simulink library "BechamoNasaOpenModels"  (R2024b)
settings: Solver=VariableStepAuto  StartTime=0.0  StopTime=10.0  RelTol=1e-3
values from neighbouring files (symbols this model uses):
  Cl_aileron_wing_1 = Cl_mat.Claileron_wing.axes1.value    [setupMavrik.m]
  Cl_aileron_wing_2 = Cl_mat.Claileron_wing.axes2.value    [setupMavrik.m]
  Cl_aileron_wing_3 = Cl_mat.Claileron_wing.axes3.value    [setupMavrik.m]
  Cl_aileron_wing_val = Cl_mat.Claileron_wing.value    [setupMavrik.m]
  Cl_elevator_tail_1 = Cl_mat.Clelevator_tail.axes1.value    [setupMavrik.m]
  Cl_elevator_tail_2 = Cl_mat.Clelevator_tail.axes2.value    [setupMavrik.m]
  Cl_elevator_tail_3 = Cl_mat.Clelevator_tail.axes3.value    [setupMavrik.m]
  Cl_elevator_tail_val = Cl_mat.Clelevator_tail.value    [setupMavrik.m]
  Cl_flap_wing_1 = Cl_mat.Clflap_wing.axes1.value    [setupMavrik.m]
  Cl_flap_wing_2 = Cl_mat.Clflap_wing.axes2.value    [setupMavrik.m]
  Cl_flap_wing_3 = Cl_mat.Clflap_wing.axes3.value    [setupMavrik.m]
  Cl_flap_wing_val = Cl_mat.Clflap_wing.value    [setupMavrik.m]
  Cl_hover_fuse_1 = Cl_mat.Clhover_fuse.axes1.value    [setupMavrik.m]
  Cl_hover_fuse_2 = Cl_mat.Clhover_fuse.axes2.value    [setupMavrik.m]
  Cl_hover_fuse_3 = Cl_mat.Clhover_fuse.axes3.value    [setupMavrik.m]
  Cl_hover_fuse_val = Cl_mat.Clhover_fuse.value    [setupMavrik.m]
  Cl_rudder_tail_1 = Cl_mat.Clrudder_tail.axes1.value    [setupMavrik.m]
  Cl_rudder_tail_2 = Cl_mat.Clrudder_tail.axes2.value    [setupMavrik.m]
  Cl_rudder_tail_3 = Cl_mat.Clrudder_tail.axes3.value    [setupMavrik.m]
  Cl_rudder_tail_val = Cl_mat.Clrudder_tail.value    [setupMavrik.m]
  Cl_tail_1 = Cl_mat.Cltail.axes1.value    [setupMavrik.m]
  Cl_tail_2 = Cl_mat.Cltail.axes2.value    [setupMavrik.m]
  Cl_tail_3 = Cl_mat.Cltail.axes3.value    [setupMavrik.m]
  Cl_tail_damp_p_1 = Cl_mat.Cltail_damp_p.axes1.value    [setupMavrik.m]
  Cl_tail_damp_p_2 = Cl_mat.Cltail_damp_p.axes2.value    [setupMavrik.m]
  Cl_tail_damp_p_3 = Cl_mat.Cltail_damp_p.axes3.value    [setupMavrik.m]
  Cl_tail_damp_p_val = Cl_mat.Cltail_damp_p.value    [setupMavrik.m]
  Cl_tail_damp_q_1 = Cl_mat.Cltail_damp_q.axes1.value    [setupMavrik.m]
  Cl_tail_damp_q_2 = Cl_mat.Cltail_damp_q.axes2.value    [setupMavrik.m]
  Cl_tail_damp_q_3 = Cl_mat.Cltail_damp_q.axes3.value    [setupMavrik.m]
  Cl_tail_damp_q_val = Cl_mat.Cltail_damp_q.value    [setupMavrik.m]
  Cl_tail_damp_r_1 = Cl_mat.Cltail_damp_r.axes1.value    [setupMavrik.m]
  Cl_tail_damp_r_2 = Cl_mat.Cltail_damp_r.axes2.value    [setupMavrik.m]
  Cl_tail_damp_r_3 = Cl_mat.Cltail_damp_r.axes3.value    [setupMavrik.m]
  Cl_tail_damp_r_val = Cl_mat.Cltail_damp_r.value    [setupMavrik.m]
  Cl_tail_val = Cl_mat.Cltail.value    [setupMavrik.m]
  Cl_wing_1 = Cl_mat.Clwing.axes1.value    [setupMavrik.m]
  Cl_wing_2 = Cl_mat.Clwing.axes2.value    [setupMavrik.m]
  Cl_wing_3 = Cl_mat.Clwing.axes3.value    [setupMavrik.m]
  Cl_wing_damp_p_1 = Cl_mat.Clwing_damp_p.axes1.value    [setupMavrik.m]
  Cl_wing_damp_p_2 = Cl_mat.Clwing_damp_p.axes2.value    [setupMavrik.m]
  Cl_wing_damp_p_3 = Cl_mat.Clwing_damp_p.axes3.value    [setupMavrik.m]
  Cl_wing_damp_p_val = Cl_mat.Clwing_damp_p.value    [setupMavrik.m]
  Cl_wing_damp_q_1 = Cl_mat.Clwing_damp_q.axes1.value    [setupMavrik.m]
  Cl_wing_damp_q_2 = Cl_mat.Clwing_damp_q.axes2.value    [setupMavrik.m]
  Cl_wing_damp_q_3 = Cl_mat.Clwing_damp_q.axes3.value    [setupMavrik.m]
  Cl_wing_damp_q_val = Cl_mat.Clwing_damp_q.value    [setupMavrik.m]
  Cl_wing_damp_r_1 = Cl_mat.Clwing_damp_r.axes1.value    [setupMavrik.m]
  Cl_wing_damp_r_2 = Cl_mat.Clwing_damp_r.axes2.value    [setupMavrik.m]
  Cl_wing_damp_r_3 = Cl_mat.Clwing_damp_r.axes3.value    [setupMavrik.m]
  Cl_wing_damp_r_val = Cl_mat.Clwing_damp_r.value    [setupMavrik.m]
  Cl_wing_val = Cl_mat.Clwing.value    [setupMavrik.m]
  Cm_aileron_wing_1 = Cm_mat.Cmaileron_wing.axes1.value    [setupMavrik.m]
  Cm_aileron_wing_2 = Cm_mat.Cmaileron_wing.axes2.value    [setupMavrik.m]
  Cm_aileron_wing_3 = Cm_mat.Cmaileron_wing.axes3.value    [setupMavrik.m]
  Cm_aileron_wing_val = Cm_mat.Cmaileron_wing.value    [setupMavrik.m]
  Cm_elevator_tail_1 = Cm_mat.Cmelevator_tail.axes1.value    [setupMavrik.m]
  Cm_elevator_tail_2 = Cm_mat.Cmelevator_tail.axes2.value    [setupMavrik.m]
  Cm_elevator_tail_3 = Cm_mat.Cmelevator_tail.axes3.value    [setupMavrik.m]
  Cm_elevator_tail_val = Cm_mat.Cmelevator_tail.value    [setupMavrik.m]
  Cm_flap_wing_1 = Cm_mat.Cmflap_wing.axes1.value    [setupMavrik.m]
  Cm_flap_wing_2 = Cm_mat.Cmflap_wing.axes2.value    [setupMavrik.m]
  Cm_flap_wing_3 = Cm_mat.Cmflap_wing.axes3.value    [setupMavrik.m]
  Cm_flap_wing_val = Cm_mat.Cmflap_wing.value    [setupMavrik.m]
  Cm_hover_fuse_1 = Cm_mat.Cmhover_fuse.axes1.value    [setupMavrik.m]
  Cm_hover_fuse_2 = Cm_mat.Cmhover_fuse.axes2.value    [setupMavrik.m]
  Cm_hover_fuse_3 = Cm_mat.Cmhover_fuse.axes3.value    [setupMavrik.m]
  Cm_hover_fuse_val = Cm_mat.Cmhover_fuse.value    [setupMavrik.m]
  Cm_rudder_tail_1 = Cm_mat.Cmrudder_tail.axes1.value    [setupMavrik.m]
  Cm_rudder_tail_2 = Cm_mat.Cmrudder_tail.axes2.value    [setupMavrik.m]
  Cm_rudder_tail_3 = Cm_mat.Cmrudder_tail.axes3.value    [setupMavrik.m]
  Cm_rudder_tail_val = Cm_mat.Cmrudder_tail.value    [setupMavrik.m]
  Cm_tail_1 = Cm_mat.Cmtail.axes1.value    [setupMavrik.m]
  Cm_tail_2 = Cm_mat.Cmtail.axes2.value    [setupMavrik.m]
  Cm_tail_3 = Cm_mat.Cmtail.axes3.value    [setupMavrik.m]
  Cm_tail_damp_p_1 = Cm_mat.Cmtail_damp_p.axes1.value    [setupMavrik.m]
  Cm_tail_damp_p_2 = Cm_mat.Cmtail_damp_p.axes2.value    [setupMavrik.m]
  Cm_tail_damp_p_3 = Cm_mat.Cmtail_damp_p.axes3.value    [setupMavrik.m]
  Cm_tail_damp_p_val = Cm_mat.Cmtail_damp_p.value    [setupMavrik.m]
  Cm_tail_damp_q_1 = Cm_mat.Cmtail_damp_q.axes1.value    [setupMavrik.m]
  Cm_tail_damp_q_2 = Cm_mat.Cmtail_damp_q.axes2.value    [setupMavrik.m]
  Cm_tail_damp_q_3 = Cm_mat.Cmtail_damp_q.axes3.value    [setupMavrik.m]
  Cm_tail_damp_q_val = Cm_mat.Cmtail_damp_q.value    [setupMavrik.m]
  Cm_tail_damp_r_1 = Cm_mat.Cmtail_damp_r.axes1.value    [setupMavrik.m]
  Cm_tail_damp_r_2 = Cm_mat.Cmtail_damp_r.axes2.value    [setupMavrik.m]
  Cm_tail_damp_r_3 = Cm_mat.Cmtail_damp_r.axes3.value    [setupMavrik.m]
  Cm_tail_damp_r_val = Cm_mat.Cmtail_damp_r.value    [setupMavrik.m]
  Cm_tail_val = Cm_mat.Cmtail.value    [setupMavrik.m]
  Cm_wing_1 = Cm_mat.Cmwing.axes1.value    [setupMavrik.m]
  Cm_wing_2 = Cm_mat.Cmwing.axes2.value    [setupMavrik.m]
  Cm_wing_3 = Cm_mat.Cmwing.axes3.value    [setupMavrik.m]
  Cm_wing_damp_p_1 = Cm_mat.Cmwing_damp_p.axes1.value    [setupMavrik.m]
  Cm_wing_damp_p_2 = Cm_mat.Cmwing_damp_p.axes2.value    [setupMavrik.m]
  Cm_wing_damp_p_3 = Cm_mat.Cmwing_damp_p.axes3.value    [setupMavrik.m]
  Cm_wing_damp_p_val = Cm_mat.Cmwing_damp_p.value    [setupMavrik.m]
  Cm_wing_damp_q_1 = Cm_mat.Cmwing_damp_q.axes1.value    [setupMavrik.m]
  Cm_wing_damp_q_2 = Cm_mat.Cmwing_damp_q.axes2.value    [setupMavrik.m]
  Cm_wing_damp_q_3 = Cm_mat.Cmwing_damp_q.axes3.value    [setupMavrik.m]
  Cm_wing_damp_q_val = Cm_mat.Cmwing_damp_q.value    [setupMavrik.m]
  Cm_wing_damp_r_1 = Cm_mat.Cmwing_damp_r.axes1.value    [setupMavrik.m]
  Cm_wing_damp_r_2 = Cm_mat.Cmwing_damp_r.axes2.value    [setupMavrik.m]
  Cm_wing_damp_r_3 = Cm_mat.Cmwing_damp_r.axes3.value    [setupMavrik.m]
  Cm_wing_damp_r_val = Cm_mat.Cmwing_damp_r.value    [setupMavrik.m]
  Cm_wing_val = Cm_mat.Cmwing.value    [setupMavrik.m]
  Cn_aileron_wing_1 = Cn_mat.Cnaileron_wing.axes1.value    [setupMavrik.m]
  Cn_aileron_wing_2 = Cn_mat.Cnaileron_wing.axes2.value    [setupMavrik.m]
  Cn_aileron_wing_3 = Cn_mat.Cnaileron_wing.axes3.value    [setupMavrik.m]
  Cn_aileron_wing_val = Cn_mat.Cnaileron_wing.value    [setupMavrik.m]
  Cn_elevator_tail_1 = Cn_mat.Cnelevator_tail.axes1.value    [setupMavrik.m]
  Cn_elevator_tail_2 = Cn_mat.Cnelevator_tail.axes2.value    [setupMavrik.m]
  Cn_elevator_tail_3 = Cn_mat.Cnelevator_tail.axes3.value    [setupMavrik.m]
  Cn_elevator_tail_val = Cn_mat.Cnelevator_tail.value    [setupMavrik.m]
  Cn_flap_wing_1 = Cn_mat.Cnflap_wing.axes1.value    [setupMavrik.m]
  Cn_flap_wing_2 = Cn_mat.Cnflap_wing.axes2.value    [setupMavrik.m]
  Cn_flap_wing_3 = Cn_mat.Cnflap_wing.axes3.value    [setupMavrik.m]
  Cn_flap_wing_val = Cn_mat.Cnflap_wing.value    [setupMavrik.m]
  Cn_hover_fuse_1 = Cn_mat.Cnhover_fuse.axes1.value    [setupMavrik.m]
  Cn_hover_fuse_2 = Cn_mat.Cnhover_fuse.axes2.value    [setupMavrik.m]
  Cn_hover_fuse_3 = Cn_mat.Cnhover_fuse.axes3.value    [setupMavrik.m]
  Cn_hover_fuse_val = Cn_mat.Cnhover_fuse.value    [setupMavrik.m]
  ... (+319 more)
libraries: matrix_library x15, sharedtransform x2, $bdroot x1, shared6dof x1
(part 16 of 19)

== matlab function BechamoNasaOpenModels/Mavrik v1/Mavrik Aero/Kq/MATLAB Function205 ==
  data: u input size=[1 45]; Wing_Transform output
function Wing_Transform = fcn(u)

% Find Interpolation Points
variable_indices = struct('U', 1, 'alpha', 2, 'beta', 3, 'p', 4, 'q', 5, 'r', 6, 'wing_alpha', 7, 'wing_beta', 8, 'wing_RPM', 9, 'left_alpha', 10,...
    'right_alpha', 11, 'left_beta', 12, 'right_beta', 13, 'wing_prop_alpha', 14, 'wing_prop_beta', 15, 'tail_alpha', 16, 'tail_beta', 17, 'tail_RPM', 18, 'tailLeft_alpha', 19, 'tailRight_alpha', 20,...
    'tailLeft_beta', 21, 'tailRight_beta', 22, 'tail_prop_alpha', 23, 'tail_prop_beta', 24, 'Q', 25, 'aileron', 26, 'elevator', 27, 'flap', 28, 'rudder', 29, 'wing_tilt', 30,...
    'tail_tilt', 31, 'RPM_tailLeft', 32, 'RPM_tailRight', 33, 'RPM_leftOut1', 34, 'RPM_left2', 35, 'RPM_left3', 36, 'RPM_left4', 37, 'RPM_left5', 38, 'RPM_left6In', 39, 'RPM_right7In', 40,...
    'RPM_right8', 41, 'RPM_right9', 42, 'RPM_right10', 43, 'RPM_right11', 44, 'RPM_right12Out', 45);

wing_tilt = u(variable_indices.wing_tilt);
Wing_Transform = [cos(wing_tilt) 0 sin(wing_tilt); 0 1 0; -sin(wing_tilt) 0 cos(wing_tilt)];

end

% y = [U, alpha, beta, p, q, r, wing_alpha, wing_beta, wing_RPM, left_alpha, right_alpha, left_beta, right_beta, wing_prop_alpha, wing_prop_beta, ...
    % tail_alpha, tail_beta, tail_RPM, tailLeft_alpha, tailRight_alpha, tailLeft_beta, tailRight_beta, tail_prop_alpha, ...
    % tail_prop_beta, Q, aileron, elevator, flap, rudder, wing_tilt, tail_tilt, RPM_tailLeft, RPM_tailRight, RPM_leftOut1, RPM_left2, ...
    % RPM_left3, RPM_left4, RPM_left5, RPM_left6In, RPM_right7In, RPM_right8, RPM_right9, RPM_right10, RPM_right11, RPM_right12Out];

== matlab function BechamoNasaOpenModels/Mavrik v1/Mavrik Aero/Cy/CY_wing_damp_p ==
  data: u input size=[1 45]; interp_point_1 output; interp_point_2 output; interp_point_3 output; interp_point_4 output; interp_point_5 output; interp_point_6 output
function [interp_point_1, interp_point_2, interp_point_3, interp_point_4, interp_point_5, interp_point_6] = fcn(u)

% Find Interpolation Points
variable_indices = struct('U', 1, 'alpha', 2, 'beta', 3, 'p', 4, 'q', 5, 'r', 6, 'wing_alpha', 7, 'wing_beta', 8, 'wing_RPM', 9, 'left_alpha', 10,...
    'right_alpha', 11, 'left_beta', 12, 'right_beta', 13, 'wing_prop_alpha', 14, 'wing_prop_beta', 15, 'tail_alpha', 16, 'tail_beta', 17, 'tail_RPM', 18, 'tailLeft_alpha', 19, 'tailRight_alpha', 20,...
    'tailLeft_beta', 21, 'tailRight_beta', 22, 'tail_prop_alpha', 23, 'tail_prop_beta', 24, 'Q', 25, 'aileron', 26, 'elevator', 27, 'flap', 28, 'rudder', 29, 'wing_tilt', 30,...
    'tail_tilt', 31, 'RPM_tailLeft', 32, 'RPM_tailRight', 33, 'RPM_leftOut1', 34, 'RPM_left2', 35, 'RPM_left3', 36, 'RPM_left4', 37, 'RPM_left5', 38, 'RPM_left6In', 39, 'RPM_right7In', 40,...
    'RPM_right8', 41, 'RPM_right9', 42, 'RPM_right10', 43, 'RPM_right11', 44, 'RPM_right12Out', 45);

interp_point_1  = u(variable_indices.wing_alpha);
interp_point_2  = u(variable_indices.wing_beta);
interp_point_3  = u(variable_indices.U);
interp_point_4  = u(variable_indices.wing_RPM);
interp_point_5  = u(variable_indices.wing_prop_alpha);
interp_point_6  = u(variable_indices.wing_prop_beta);

end

% y = [U, alpha, beta, p, q, r, wing_alpha, wing_beta, wing_RPM, left_alpha, right_alpha, left_beta, right_beta, wing_prop_alpha, wing_prop_beta, ...
    % tail_alpha, tail_beta, tail_RPM, tailLeft_alpha, tailRight_alpha, tailLeft_beta, tailRight_beta, tail_prop_alpha, ...
    % tail_prop_beta, Q, aileron, elevator, flap, rudder, wing_tilt, tail_tilt, RPM_tailLeft, RPM_tailRight, RPM_leftOut1, RPM_left2, ...
    % RPM_left3, RPM_left4, RPM_left5, RPM_left6In, RPM_right7In, RPM_right8, RPM_right9, RPM_right10, RPM_right11, RPM_right12Out];

== matlab function BechamoNasaOpenModels/Mavrik v1/Mavrik Aero/Cy/CY_wing_damp_q ==
  data: u input size=[1 45]; interp_point_1 output; interp_point_2 output; interp_point_3 output; interp_point_4 output; interp_point_5 output; interp_point_6 output
function [interp_point_1, interp_point_2, interp_point_3, interp_point_4, interp_point_5, interp_point_6] = fcn(u)

% Find Interpolation Points
variable_indices = struct('U', 1, 'alpha', 2, 'beta', 3, 'p', 4, 'q', 5, 'r', 6, 'wing_alpha', 7, 'wing_beta', 8, 'wing_RPM', 9, 'left_alpha', 10,...
    'right_alpha', 11, 'left_beta', 12, 'right_beta', 13, 'wing_prop_alpha', 14, 'wing_prop_beta', 15, 'tail_alpha', 16, 'tail_beta', 17, 'tail_RPM', 18, 'tailLeft_alpha', 19, 'tailRight_alpha', 20,...
    'tailLeft_beta', 21, 'tailRight_beta', 22, 'tail_prop_alpha', 23, 'tail_prop_beta', 24, 'Q', 25, 'aileron', 26, 'elevator', 27, 'flap', 28, 'rudder', 29, 'wing_tilt', 30,...
    'tail_tilt', 31, 'RPM_tailLeft', 32, 'RPM_tailRight', 33, 'RPM_leftOut1', 34, 'RPM_left2', 35, 'RPM_left3', 36, 'RPM_left4', 37, 'RPM_left5', 38, 'RPM_left6In', 39, 'RPM_right7In', 40,...
    'RPM_right8', 41, 'RPM_right9', 42, 'RPM_right10', 43, 'RPM_right11', 44, 'RPM_right12Out', 45);

interp_point_1  = u(variable_indices.wing_alpha);
interp_point_2  = u(variable_indices.wing_beta);
interp_point_3  = u(variable_indices.U);
interp_point_4  = u(variable_indices.wing_RPM);
interp_point_5  = u(variable_indices.wing_prop_alpha);
interp_point_6  = u(variable_indices.wing_prop_beta);

end

% y = [U, alpha, beta, p, q, r, wing_alpha, wing_beta, wing_RPM, left_alpha, right_alpha, left_beta, right_beta, wing_prop_alpha, wing_prop_beta, ...
    % tail_alpha, tail_beta, tail_RPM, tailLeft_alpha, tailRight_alpha, tailLeft_beta, tailRight_beta, tail_prop_alpha, ...
    % tail_prop_beta, Q, aileron, elevator, flap, rudder, wing_tilt, tail_tilt, RPM_tailLeft, RPM_tailRight, RPM_leftOut1, RPM_left2, ...
    % RPM_left3, RPM_left4, RPM_left5, RPM_left6In, RPM_right7In, RPM_right8, RPM_right9, RPM_right10, RPM_right11, RPM_right12Out];

== matlab function BechamoNasaOpenModels/Mavrik v1/Mavrik Aero/Function Block 1 ==
  data: u input size=[1 9]; y output size=[1 45]; actuators input
function y  = fcn(u, actuators)

% Setup input states
U = sqrt(u(1)^2+u(2)^2+u(3)^2);
alpha = atan2(u(3), u(1));
beta = atan2(u(2),sqrt(u(1)^2+u(3)^2));
p = u(4);
q = u(5);
r = u(6);
phi = u(7);
theta = u(8);
psi = u(9);

rho = 1.225;

% Actuation Inputs
wing_tilt = actuators(1);
tail_tilt = actuators(2); 
aileron = actuators(3);
elevator = actuators(4);
flap = actuators(5);
rudder = actuators(6);
RPM_tailLeft = actuators(7);
RPM_tailRight = actuators(8);
RPM_leftOut1 = actuators(9);
RPM_left2 = actuators(10);
RPM_left3 = actuators(11);
RPM_left4 = actuators(12);
RPM_left5 = actuators(13);
RPM_left6In = actuators(14);
RPM_right7In = actuators(15);
RPM_right8 = actuators(16);
RPM_right9 = actuators(17);
RPM_right10 = actuators(18);
RPM_right11 = actuators(19);
RPM_right12Out = actuators(20);

% Calculate alpha/beta for local tables

wing_alpha = alpha + wing_tilt;
wing_beta = beta;
wing_RPM = 1/12 * (RPM_leftOut1 + RPM_left2 + RPM_left3 + RPM_left4 + RPM_left5 + RPM_left6In + RPM_right7In + RPM_right8 + RPM_right9 + RPM_right10 + RPM_right11 + RPM_right12Out);
left_alpha = alpha + wing_tilt; 
right_alpha = alpha + wing_tilt;
left_beta = beta;
right_beta = beta;
wing_prop_alpha = 1/2 * sum(left_alpha + right_alpha);
wing_prop_beta = 1/2 * sum(left_beta + right_beta);
tail_alpha = alpha + tail_tilt;
tail_beta = beta;
tail_RPM = 0.5 * (RPM_tailRight + RPM_tailLeft); 
tailLeft_alpha = alpha + tail_tilt;
tailRight_alpha = alpha + tail_tilt; 
tailLeft_beta = beta;
tailRight_beta = beta; 
tail_prop_alpha = 0.5 * (tailLeft_alpha + tailRight_alpha);
tail_prop_beta = 0.5 * (tailLeft_beta + tailRight_beta); 
Q = 0.5*rho*U^2;

y = [U, alpha, beta, p, q, r, wing_alpha, wing_beta, wing_RPM, left_alpha, right_alpha, left_beta, right_beta, wing_prop_alpha, wing_prop_beta, ...
    tail_alpha, tail_beta, tail_RPM, tailLeft_alpha, tailRight_alpha, tailLeft_beta, tailRight_beta, tail_prop_alpha, ...
    tail_prop_beta, Q, aileron, elevator, flap, rudder, wing_tilt, tail_tilt, RPM_tailLeft, RPM_tailRight, RPM_leftOut1, RPM_left2, ...
    RPM_left3, RPM_left4, RPM_left5, RPM_left6In, RPM_right7In, RPM_right8, RPM_right9, RPM_right10, RPM_right11, RPM_right12Out];

end

== matlab function BechamoNasaOpenModels/Mavrik v1/Mavrik Aero/Cy/CY_wing_damp_r ==
  data: u input size=[1 45]; interp_point_1 output; interp_point_2 output; interp_point_3 output; interp_point_4 output; interp_point_5 output; interp_point_6 output
function [interp_point_1, interp_point_2, interp_point_3, interp_point_4, interp_point_5, interp_point_6] = fcn(u)

% Find Interpolation Points
variable_indices = struct('U', 1, 'alpha', 2, 'beta', 3, 'p', 4, 'q', 5, 'r', 6, 'wing_alpha', 7, 'wing_beta', 8, 'wing_RPM', 9, 'left_alpha', 10,...
    'right_alpha', 11, 'left_beta', 12, 'right_beta', 13, 'wing_prop_alpha', 14, 'wing_prop_beta', 15, 'tail_alpha', 16, 'tail_beta', 17, 'tail_RPM', 18, 'tailLeft_alpha', 19, 'tailRight_alpha', 20,...
    'tailLeft_beta', 21, 'tailRight_beta', 22, 'tail_prop_alpha', 23, 'tail_prop_beta', 24, 'Q', 25, 'aileron', 26, 'elevator', 27, 'flap', 28, 'rudder', 29, 'wing_tilt', 30,...
    'tail_tilt', 31, 'RPM_tailLeft', 32, 'RPM_tailRight', 33, 'RPM_leftOut1', 34, 'RPM_left2', 35, 'RPM_left3', 36, 'RPM_left4', 37, 'RPM_left5', 38, 'RPM_left6In', 39, 'RPM_right7In', 40,...
    'RPM_right8', 41, 'RPM_right9', 42, 'RPM_right10', 43, 'RPM_right11', 44, 'RPM_right12Out', 45);

interp_point_1  = u(variable_indices.wing_alpha);
interp_point_2  = u(variable_indices.wing_beta);
interp_point_3  = u(variable_indices.U);
interp_point_4  = u(variable_indices.wing_RPM);
interp_point_5  = u(variable_indices.wing_prop_alpha);
interp_point_6  = u(variable_indices.wing_prop_beta);

end

% y = [U, alpha, beta, p, q, r, wing_alpha, wing_beta, wing_RPM, left_alpha, right_alpha, left_beta, right_beta, wing_prop_alpha, wing_prop_beta, ...
    % tail_alpha, tail_beta, tail_RPM, tailLeft_alpha, tailRight_alpha, tailLeft_beta, tailRight_beta, tail_prop_alpha, ...
    % tail_prop_beta, Q, aileron, elevator, flap, rudder, wing_tilt, tail_tilt, RPM_tailLeft, RPM_tailRight, RPM_leftOut1, RPM_left2, ...
    % RPM_left3, RPM_left4, RPM_left5, RPM_left6In, RPM_right7In, RPM_right8, RPM_right9, RPM_right10, RPM_right11, RPM_right12Out];

== matlab function BechamoNasaOpenModels/Mavrik v1/Mavrik Aero/Cz/CZ_aileron_wing ==
  data: u input size=[1 45]; interp_point_1 output; interp_point_2 output; interp_point_3 output; interp_point_4 output; interp_point_5 output; interp_point_6 output; interp_point_7 output
function [interp_point_1, interp_point_2, interp_point_3, interp_point_4, interp_point_5, interp_point_6, interp_point_7] = fcn(u)

% Find Interpolation Points
variable_indices = struct('U', 1, 'alpha', 2, 'beta', 3, 'p', 4, 'q', 5, 'r', 6, 'wing_alpha', 7, 'wing_beta', 8, 'wing_RPM', 9, 'left_alpha', 10,...
    'right_alpha', 11, 'left_beta', 12, 'right_beta', 13, 'wing_prop_alpha', 14, 'wing_prop_beta', 15, 'tail_alpha', 16, 'tail_beta', 17, 'tail_RPM', 18, 'tailLeft_alpha', 19, 'tailRight_alpha', 20,...
    'tailLeft_beta', 21, 'tailRight_beta', 22, 'tail_prop_alpha', 23, 'tail_prop_beta', 24, 'Q', 25, 'aileron', 26, 'elevator', 27, 'flap', 28, 'rudder', 29, 'wing_tilt', 30,...
    'tail_tilt', 31, 'RPM_tailLeft', 32, 'RPM_tailRight', 33, 'RPM_leftOut1', 34, 'RPM_left2', 35, 'RPM_left3', 36, 'RPM_left4', 37, 'RPM_left5', 38, 'RPM_left6In', 39, 'RPM_right7In', 40,...
    'RPM_right8', 41, 'RPM_right9', 42, 'RPM_right10', 43, 'RPM_right11', 44, 'RPM_right12Out', 45);

interp_point_1  = u(variable_indices.wing_alpha);
interp_point_2  = u(variable_indices.wing_beta);
interp_point_3  = u(variable_indices.U);
interp_point_4  = u(variable_indices.wing_RPM);
interp_point_5  = u(variable_indices.wing_prop_alpha);
interp_point_6  = u(variable_indices.wing_prop_beta);
interp_point_7  = u(variable_indices.aileron);

end

% y = [U, alpha, beta, p, q, r, wing_alpha, wing_beta, wing_RPM, left_alpha, right_alpha, left_beta, right_beta, wing_prop_alpha, wing_prop_beta, ...
    % tail_alpha, tail_beta, tail_RPM, tailLeft_alpha, tailRight_alpha, tailLeft_beta, tailRight_beta, tail_prop_alpha, ...
    % tail_prop_beta, Q, aileron, elevator, flap, rudder, wing_tilt, tail_tilt, RPM_tailLeft, RPM_tailRight, RPM_leftOut1, RPM_left2, ...
    % RPM_left3, RPM_left4, RPM_left5, RPM_left6In, RPM_right7In, RPM_right8, RPM_right9, RPM_right10, RPM_right11, RPM_right12Out];

== matlab function BechamoNasaOpenModels/Mavrik v1/Mavrik Aero/Cz/CZ_elevator_tail ==
  data: u input size=[1 45]; interp_point_1 output; interp_point_2 output; interp_point_3 output; interp_point_4 output; interp_point_5 output; interp_point_6 output; interp_point_7 output
function [interp_point_1, interp_point_2, interp_point_3, interp_point_4, interp_point_5, interp_point_6, interp_point_7] = fcn(u)

% Find Interpolation Points
variable_indices = struct('U', 1, 'alpha', 2, 'beta', 3, 'p', 4, 'q', 5, 'r', 6, 'wing_alpha', 7, 'wing_beta', 8, 'wing_RPM', 9, 'left_alpha', 10,...
    'right_alpha', 11, 'left_beta', 12, 'right_beta', 13, 'wing_prop_alpha', 14, 'wing_prop_beta', 15, 'tail_alpha', 16, 'tail_beta', 17, 'tail_RPM', 18, 'tailLeft_alpha', 19, 'tailRight_alpha', 20,...
    'tailLeft_beta', 21, 'tailRight_beta', 22, 'tail_prop_alpha', 23, 'tail_prop_beta', 24, 'Q', 25, 'aileron', 26, 'elevator', 27, 'flap', 28, 'rudder', 29, 'wing_tilt', 30,...
    'tail_tilt', 31, 'RPM_tailLeft', 32, 'RPM_tailRight', 33, 'RPM_leftOut1', 34, 'RPM_left2', 35, 'RPM_left3', 36, 'RPM_left4', 37, 'RPM_left5', 38, 'RPM_left6In', 39, 'RPM_right7In', 40,...
    'RPM_right8', 41, 'RPM_right9', 42, 'RPM_right10', 43, 'RPM_right11', 44, 'RPM_right12Out', 45);

interp_point_1  = u(variable_indices.tail_alpha);
interp_point_2  = u(variable_indices.tail_beta);
interp_point_3  = u(variable_indices.U);
interp_point_4  = u(variable_indices.tail_RPM);
interp_point_5  = u(variable_indices.tail_prop_alpha);
interp_point_6  = u(variable_indices.tail_prop_beta);
interp_point_7  = u(variable_indices.elevator);

end

% y = [U, alpha, beta, p, q, r, wing_alpha, wing_beta, wing_RPM, left_alpha, right_alpha, left_beta, right_beta, wing_prop_alpha, wing_prop_beta, ...
    % tail_alpha, tail_beta, tail_RPM, tailLeft_alpha, tailRight_alpha, tailLeft_beta, tailRight_beta, tail_prop_alpha, ...
    % tail_prop_beta, Q, aileron, elevator, flap, rudder, wing_tilt, tail_tilt, RPM_tailLeft, RPM_tailRight, RPM_leftOut1, RPM_left2, ...
    % RPM_left3, RPM_left4, RPM_left5, RPM_left6In, RPM_right7In, RPM_right8, RPM_right9, RPM_right10, RPM_right11, RPM_right12Out];

== matlab function BechamoNasaOpenModels/Mavrik v1/Mavrik Aero/Cz/CZ_flap_wing ==
  data: u input size=[1 45]; interp_point_1 output; interp_point_2 output; interp_point_3 output; interp_point_4 output; interp_point_5 output; interp_point_6 output; interp_point_7 output
function [interp_point_1, interp_point_2, interp_point_3, interp_point_4, interp_point_5, interp_point_6, interp_point_7] = fcn(u)

% Find Interpolation Points
variable_indices = struct('U', 1, 'alpha', 2, 'beta', 3, 'p', 4, 'q', 5, 'r', 6, 'wing_alpha', 7, 'wing_beta', 8, 'wing_RPM', 9, 'left_alpha', 10,...
    'right_alpha', 11, 'left_beta', 12, 'right_beta', 13, 'wing_prop_alpha', 14, 'wing_prop_beta', 15, 'tail_alpha', 16, 'tail_beta', 17, 'tail_RPM', 18, 'tailLeft_alpha', 19, 'tailRight_alpha', 20,...
    'tailLeft_beta', 21, 'tailRight_beta', 22, 'tail_prop_alpha', 23, 'tail_prop_beta', 24, 'Q', 25, 'aileron', 26, 'elevator', 27, 'flap', 28, 'rudder', 29, 'wing_tilt', 30,...
    'tail_tilt', 31, 'RPM_tailLeft', 32, 'RPM_tailRight', 33, 'RPM_leftOut1', 34, 'RPM_left2', 35, 'RPM_left3', 36, 'RPM_left4', 37, 'RPM_left5', 38, 'RPM_left6In', 39, 'RPM_right7In', 40,...
    'RPM_right8', 41, 'RPM_right9', 42, 'RPM_right10', 43, 'RPM_right11', 44, 'RPM_right12Out', 45);

interp_point_1  = u(variable_indices.wing_alpha);
interp_point_2  = u(variable_indices.wing_beta);
interp_point_3  = u(variable_indices.U);
interp_point_4  = u(variable_indices.wing_RPM);
interp_point_5  = u(variable_indices.wing_prop_alpha);
interp_point_6  = u(variable_indices.wing_prop_beta);
interp_point_7  = u(variable_indices.flap);

end

% y = [U, alpha, beta, p, q, r, wing_alpha, wing_beta, wing_RPM, left_alpha, right_alpha, left_beta, right_beta, wing_prop_alpha, wing_prop_beta, ...
    % tail_alpha, tail_beta, tail_RPM, tailLeft_alpha, tailRight_alpha, tailLeft_beta, tailRight_beta, tail_prop_alpha, ...
    % tail_prop_beta, Q, aileron, elevator, flap, rudder, wing_tilt, tail_tilt, RPM_tailLeft, RPM_tailRight, RPM_leftOut1, RPM_left2, ...
    % RPM_left3, RPM_left4, RPM_left5, RPM_left6In, RPM_right7In, RPM_right8, RPM_right9, RPM_right10, RPM_right11, RPM_right12Out];

== matlab function BechamoNasaOpenModels/Mavrik v1/Mavrik Aero/Cz/CZ_rudder_tail ==
  data: u input size=[1 45]; interp_point_1 output; interp_point_2 output; interp_point_3 output; interp_point_4 output; interp_point_5 output; interp_point_6 output; interp_point_7 output
function [interp_point_1, interp_point_2, interp_point_3, interp_point_4, interp_point_5, interp_point_6, interp_point_7] = fcn(u)

% Find Interpolation Points
variable_indices = struct('U', 1, 'alpha', 2, 'beta', 3, 'p', 4, 'q', 5, 'r', 6, 'wing_alpha', 7, 'wing_beta', 8, 'wing_RPM', 9, 'left_alpha', 10,...
    'right_alpha', 11, 'left_beta', 12, 'right_beta', 13, 'wing_prop_alpha', 14, 'wing_prop_beta', 15, 'tail_alpha', 16, 'tail_beta', 17, 'tail_RPM', 18, 'tailLeft_alpha', 19, 'tailRight_alpha', 20,...
    'tailLeft_beta', 21, 'tailRight_beta', 22, 'tail_prop_alpha', 23, 'tail_prop_beta', 24, 'Q', 25, 'aileron', 26, 'elevator', 27, 'flap', 28, 'rudder', 29, 'wing_tilt', 30,...
    'tail_tilt', 31, 'RPM_tailLeft', 32, 'RPM_tailRight', 33, 'RPM_leftOut1', 34, 'RPM_left2', 35, 'RPM_left3', 36, 'RPM_left4', 37, 'RPM_left5', 38, 'RPM_left6In', 39, 'RPM_right7In', 40,...
    'RPM_right8', 41, 'RPM_right9', 42, 'RPM_right10', 43, 'RPM_right11', 44, 'RPM_right12Out', 45);

interp_point_1  = u(variable_indices.tail_alpha);
interp_point_2  = u(variable_indices.tail_beta);
interp_point_3  = u(variable_indices.U);
interp_point_4  = u(variable_indices.tail_RPM);
interp_point_5  = u(variable_indices.tail_prop_alpha);
interp_point_6  = u(variable_indices.tail_prop_beta);
interp_point_7  = u(variable_indices.rudder);

end

% y = [U, alpha, beta, p, q, r, wing_alpha, wing_beta, wing_RPM, left_alpha, right_alpha, left_beta, right_beta, wing_prop_alpha, wing_prop_beta, ...
    % tail_alpha, tail_beta, tail_RPM, tailLeft_alpha, tailRight_alpha, tailLeft_beta, tailRight_beta, tail_prop_alpha, ...
    % tail_prop_beta, Q, aileron, elevator, flap, rudder, wing_tilt, tail_tilt, RPM_tailLeft, RPM_tailRight, RPM_leftOut1, RPM_left2, ...
    % RPM_left3, RPM_left4, RPM_left5, RPM_left6In, RPM_right7In, RPM_right8, RPM_right9, RPM_right10, RPM_right11, RPM_right12Out];

== matlab function BechamoNasaOpenModels/Mavrik v1/Mavrik Aero/Cz/CZ_tail ==
  data: u input size=[1 45]; interp_point_1 output; interp_point_2 output; interp_point_3 output; interp_point_4 output; interp_point_5 output; interp_point_6 output
function [interp_point_1, interp_point_2, interp_point_3, interp_point_4, interp_point_5, interp_point_6] = fcn(u)

% Find Interpolation Points
variable_indices = struct('U', 1, 'alpha', 2, 'beta', 3, 'p', 4, 'q', 5, 'r', 6, 'wing_alpha', 7, 'wing_beta', 8, 'wing_RPM', 9, 'left_alpha', 10,...
    'right_alpha', 11, 'left_beta', 12, 'right_beta', 13, 'wing_prop_alpha', 14, 'wing_prop_beta', 15, 'tail_alpha', 16, 'tail_beta', 17, 'tail_RPM', 18, 'tailLeft_alpha', 19, 'tailRight_alpha', 20,...
    'tailLeft_beta', 21, 'tailRight_beta', 22, 'tail_prop_alpha', 23, 'tail_prop_beta', 24, 'Q', 25, 'aileron', 26, 'elevator', 27, 'flap', 28, 'rudder', 29, 'wing_tilt', 30,...
    'tail_tilt', 31, 'RPM_tailLeft', 32, 'RPM_tailRight', 33, 'RPM_leftOut1', 34, 'RPM_left2', 35, 'RPM_left3', 36, 'RPM_left4', 37, 'RPM_left5', 38, 'RPM_left6In', 39, 'RPM_right7In', 40,...
    'RPM_right8', 41, 'RPM_right9', 42, 'RPM_right10', 43, 'RPM_right11', 44, 'RPM_right12Out', 45);

interp_point_1  = u(variable_indices.tail_alpha);
interp_point_2  = u(variable_indices.tail_beta);
interp_point_3  = u(variable_indices.U);
interp_point_4  = u(variable_indices.tail_RPM);
interp_point_5  = u(variable_indices.tail_prop_alpha);
interp_point_6  = u(variable_indices.tail_prop_beta);

end

% y = [U, alpha, beta, p, q, r, wing_alpha, wing_beta, wing_RPM, left_alpha, right_alpha, left_beta, right_beta, wing_prop_alpha, wing_prop_beta, ...
    % tail_alpha, tail_beta, tail_RPM, tailLeft_alpha, tailRight_alpha, tailLeft_beta, tailRight_beta, tail_prop_alpha, ...
    % tail_prop_beta, Q, aileron, elevator, flap, rudder, wing_tilt, tail_tilt, RPM_tailLeft, RPM_tailRight, RPM_leftOut1, RPM_left2, ...
    % RPM_left3, RPM_left4, RPM_left5, RPM_left6In, RPM_right7In, RPM_right8, RPM_right9, RPM_right10, RPM_right11, RPM_right12Out];

== matlab function BechamoNasaOpenModels/Mavrik v1/Mavrik Aero/Cx/CX_aileron_wing ==
  data: u input size=[1 45]; interp_point_1 output; interp_point_2 output; interp_point_3 output; interp_point_4 output; interp_point_5 output; interp_point_6 output; interp_point_7 output
function [interp_point_1, interp_point_2, interp_point_3, interp_point_4, interp_point_5, interp_point_6, interp_point_7] = fcn(u)

% Find Interpolation Points
variable_indices = struct('U', 1, 'alpha', 2, 'beta', 3, 'p', 4, 'q', 5, 'r', 6, 'wing_alpha', 7, 'wing_beta', 8, 'wing_RPM', 9, 'left_alpha', 10,...
    'right_alpha', 11, 'left_beta', 12, 'right_beta', 13, 'wing_prop_alpha', 14, 'wing_prop_beta', 15, 'tail_alpha', 16, 'tail_beta', 17, 'tail_RPM', 18, 'tailLeft_alpha', 19, 'tailRight_alpha', 20,...
    'tailLeft_beta', 21, 'tailRight_beta', 22, 'tail_prop_alpha', 23, 'tail_prop_beta', 24, 'Q', 25, 'aileron', 26, 'elevator', 27, 'flap', 28, 'rudder', 29, 'wing_tilt', 30,...
    'tail_tilt', 31, 'RPM_tailLeft', 32, 'RPM_tailRight', 33, 'RPM_leftOut1', 34, 'RPM_left2', 35, 'RPM_left3', 36, 'RPM_left4', 37, 'RPM_left5', 38, 'RPM_left6In', 39, 'RPM_right7In', 40,...
    'RPM_right8', 41, 'RPM_right9', 42, 'RPM_right10', 43, 'RPM_right11', 44, 'RPM_right12Out', 45);

interp_point_1  = u(variable_indices.wing_alpha);
interp_point_2  = u(variable_indices.wing_beta);
interp_point_3  = u(variable_indices.U);
interp_point_4  = u(variable_indices.wing_RPM);
interp_point_5  = u(variable_indices.wing_prop_alpha);
interp_point_6  = u(variable_indices.wing_prop_beta);
interp_point_7  = u(variable_indices.aileron);

end

% y = [U, alpha, beta, p, q, r, wing_alpha, wing_beta, wing_RPM, left_alpha, right_alpha, left_beta, right_beta, wing_prop_alpha, wing_prop_beta, ...
    % tail_alpha, tail_beta, tail_RPM, tailLeft_alpha, tailRight_alpha, tailLeft_beta, tailRight_beta, tail_prop_alpha, ...
    % tail_prop_beta, Q, aileron, elevator, flap, rudder, wing_tilt, tail_tilt, RPM_tailLeft, RPM_tailRight, RPM_leftOut1, RPM_left2, ...
    % RPM_left3, RPM_left4, RPM_left5, RPM_left6In, RPM_right7In, RPM_right8, RPM_right9, RPM_right10, RPM_right11, RPM_right12Out];

== matlab function BechamoNasaOpenModels/Mavrik v1/Mavrik Aero/Cz/CZ_tail_damp_p ==
  data: u input size=[1 45]; interp_point_1 output; interp_point_2 output; interp_point_3 output; interp_point_4 output; interp_point_5 output; interp_point_6 output
function [interp_point_1, interp_point_2, interp_point_3, interp_point_4, interp_point_5, interp_point_6] = fcn(u)

% Find Interpolation Points
variable_indices = struct('U', 1, 'alpha', 2, 'beta', 3, 'p', 4, 'q', 5, 'r', 6, 'wing_alpha', 7, 'wing_beta', 8, 'wing_RPM', 9, 'left_alpha', 10,...
    'right_alpha', 11, 'left_beta', 12, 'right_beta', 13, 'wing_prop_alpha', 14, 'wing_prop_beta', 15, 'tail_alpha', 16, 'tail_beta', 17, 'tail_RPM', 18, 'tailLeft_alpha', 19, 'tailRight_alpha', 20,...
    'tailLeft_beta', 21, 'tailRight_beta', 22, 'tail_prop_alpha', 23, 'tail_prop_beta', 24, 'Q', 25, 'aileron', 26, 'elevator', 27, 'flap', 28, 'rudder', 29, 'wing_tilt', 30,...
    'tail_tilt', 31, 'RPM_tailLeft', 32, 'RPM_tailRight', 33, 'RPM_leftOut1', 34, 'RPM_left2', 35, 'RPM_left3', 36, 'RPM_left4', 37, 'RPM_left5', 38, 'RPM_left6In', 39, 'RPM_right7In', 40,...
    'RPM_right8', 41, 'RPM_right9', 42, 'RPM_right10', 43, 'RPM_right11', 44, 'RPM_right12Out', 45);

interp_point_1  = u(variable_indices.tail_alpha);
interp_point_2  = u(variable_indices.tail_beta);
interp_point_3  = u(variable_indices.U);
interp_point_4  = u(variable_indices.tail_RPM);
interp_point_5  = u(variable_indices.tail_prop_alpha);
interp_point_6  = u(variable_indices.tail_prop_beta);

end

% y = [U, alpha, beta, p, q, r, wing_alpha, wing_beta, wing_RPM, left_alpha, right_alpha, left_beta, right_beta, wing_prop_alpha, wing_prop_beta, ...
    % tail_alpha, tail_beta, tail_RPM, tailLeft_alpha, tailRight_alpha, tailLeft_beta, tailRight_beta, tail_prop_alpha, ...
    % tail_prop_beta, Q, aileron, elevator, flap, rudder, wing_tilt, tail_tilt, RPM_tailLeft, RPM_tailRight, RPM_leftOut1, RPM_left2, ...
    % RPM_left3, RPM_left4, RPM_left5, RPM_left6In, RPM_right7In, RPM_right8, RPM_right9, RPM_right10, RPM_right11, RPM_right12Out];

== matlab function BechamoNasaOpenModels/Mavrik v1/Mavrik Aero/Cz/CZ_tail_damp_q ==
  data: u input size=[1 45]; interp_point_1 output; interp_point_2 output; interp_point_3 output; interp_point_4 output; interp_point_5 output; interp_point_6 output
function [interp_point_1, interp_point_2, interp_point_3, interp_point_4, interp_point_5, interp_point_6] = fcn(u)

% Find Interpolation Points
variable_indices = struct('U', 1, 'alpha', 2, 'beta', 3, 'p', 4, 'q', 5, 'r', 6, 'wing_alpha', 7, 'wing_beta', 8, 'wing_RPM', 9, 'left_alpha', 10,...
    'right_alpha', 11, 'left_beta', 12, 'right_beta', 13, 'wing_prop_alpha', 14, 'wing_prop_beta', 15, 'tail_alpha', 16, 'tail_beta', 17, 'tail_RPM', 18, 'tailLeft_alpha', 19, 'tailRight_alpha', 20,...
    'tailLeft_beta', 21, 'tailRight_beta', 22, 'tail_prop_alpha', 23, 'tail_prop_beta', 24, 'Q', 25, 'aileron', 26, 'elevator', 27, 'flap', 28, 'rudder', 29, 'wing_tilt', 30,...
    'tail_tilt', 31, 'RPM_tailLeft', 32, 'RPM_tailRight', 33, 'RPM_leftOut1', 34, 'RPM_left2', 35, 'RPM_left3', 36, 'RPM_left4', 37, 'RPM_left5', 38, 'RPM_left6In', 39, 'RPM_right7In', 40,...
    'RPM_right8', 41, 'RPM_right9', 42, 'RPM_right10', 43, 'RPM_right11', 44, 'RPM_right12Out', 45);

interp_point_1  = u(variable_indices.tail_alpha);
interp_point_2  = u(variable_indices.tail_beta);
interp_point_3  = u(variable_indices.U);
interp_point_4  = u(variable_indices.tail_RPM);
interp_point_5  = u(variable_indices.tail_prop_alpha);
interp_point_6  = u(variable_indices.tail_prop_beta);

end

% y = [U, alpha, beta, p, q, r, wing_alpha, wing_beta, wing_RPM, left_alpha, right_alpha, left_beta, right_beta, wing_prop_alpha, wing_prop_beta, ...
    % tail_alpha, tail_beta, tail_RPM, tailLeft_alpha, tailRight_alpha, tailLeft_beta, tailRight_beta, tail_prop_alpha, ...
    % tail_prop_beta, Q, aileron, elevator, flap, rudder, wing_tilt, tail_tilt, RPM_tailLeft, RPM_tailRight, RPM_leftOut1, RPM_left2, ...
    % RPM_left3, RPM_left4, RPM_left5, RPM_left6In, RPM_right7In, RPM_right8, RPM_right9, RPM_right10, RPM_right11, RPM_right12Out];

== matlab function BechamoNasaOpenModels/Mavrik v1/Mavrik Aero/Cz/CZ_tail_damp_r ==
  data: u input size=[1 45]; interp_point_1 output; interp_point_2 output; interp_point_3 output; interp_point_4 output; interp_point_5 output; interp_point_6 output
function [interp_point_1, interp_point_2, interp_point_3, interp_point_4, interp_point_5, interp_point_6] = fcn(u)

% Find Interpolation Points
variable_indices = struct('U', 1, 'alpha', 2, 'beta', 3, 'p', 4, 'q', 5, 'r', 6, 'wing_alpha', 7, 'wing_beta', 8, 'wing_RPM', 9, 'left_alpha', 10,...
    'right_alpha', 11, 'left_beta', 12, 'right_beta', 13, 'wing_prop_alpha', 14, 'wing_prop_beta', 15, 'tail_alpha', 16, 'tail_beta', 17, 'tail_RPM', 18, 'tailLeft_alpha', 19, 'tailRight_alpha', 20,...
    'tailLeft_beta', 21, 'tailRight_beta', 22, 'tail_prop_alpha', 23, 'tail_prop_beta', 24, 'Q', 25, 'aileron', 26, 'elevator', 27, 'flap', 28, 'rudder', 29, 'wing_tilt', 30,...
    'tail_tilt', 31, 'RPM_tailLeft', 32, 'RPM_tailRight', 33, 'RPM_leftOut1', 34, 'RPM_left2', 35, 'RPM_left3', 36, 'RPM_left4', 37, 'RPM_left5', 38, 'RPM_left6In', 39, 'RPM_right7In', 40,...
    'RPM_right8', 41, 'RPM_right9', 42, 'RPM_right10', 43, 'RPM_right11', 44, 'RPM_right12Out', 45);

interp_point_1  = u(variable_indices.tail_alpha);
interp_point_2  = u(variable_indices.tail_beta);
interp_point_3  = u(variable_indices.U);
interp_point_4  = u(variable_indices.tail_RPM);
interp_point_5  = u(variable_indices.tail_prop_alpha);
interp_point_6  = u(variable_indices.tail_prop_beta);

end

% y = [U, alpha, beta, p, q, r, wing_alpha, wing_beta, wing_RPM, left_alpha, right_alpha, left_beta, right_beta, wing_prop_alpha, wing_prop_beta, ...
    % tail_alpha, tail_beta, tail_RPM, tailLeft_alpha, tailRight_alpha, tailLeft_beta, tailRight_beta, tail_prop_alpha, ...
    % tail_prop_beta, Q, aileron, elevator, flap, rudder, wing_tilt, tail_tilt, RPM_tailLeft, RPM_tailRight, RPM_leftOut1, RPM_left2, ...
    % RPM_left3, RPM_left4, RPM_left5, RPM_left6In, RPM_right7In, RPM_right8, RPM_right9, RPM_right10, RPM_right11, RPM_right12Out];

== matlab function BechamoNasaOpenModels/Mavrik v1/Mavrik Aero/Cz/CZ_wing ==
  data: u input size=[1 45]; interp_point_1 output; interp_point_2 output; interp_point_3 output; interp_point_4 output; interp_point_5 output; interp_point_6 output
function [interp_point_1, interp_point_2, interp_point_3, interp_point_4, interp_point_5, interp_point_6] = fcn(u)

% Find Interpolation Points
variable_indices = struct('U', 1, 'alpha', 2, 'beta', 3, 'p', 4, 'q', 5, 'r', 6, 'wing_alpha', 7, 'wing_beta', 8, 'wing_RPM', 9, 'left_alpha', 10,...
    'right_alpha', 11, 'left_beta', 12, 'right_beta', 13, 'wing_prop_alpha', 14, 'wing_prop_beta', 15, 'tail_alpha', 16, 'tail_beta', 17, 'tail_RPM', 18, 'tailLeft_alpha', 19, 'tailRight_alpha', 20,...
    'tailLeft_beta', 21, 'tailRight_beta', 22, 'tail_prop_alpha', 23, 'tail_prop_beta', 24, 'Q', 25, 'aileron', 26, 'elevator', 27, 'flap', 28, 'rudder', 29, 'wing_tilt', 30,...
    'tail_tilt', 31, 'RPM_tailLeft', 32, 'RPM_tailRight', 33, 'RPM_leftOut1', 34, 'RPM_left2', 35, 'RPM_left3', 36, 'RPM_left4', 37, 'RPM_left5', 38, 'RPM_left6In', 39, 'RPM_right7In', 40,...
    'RPM_right8', 41, 'RPM_right9', 42, 'RPM_right10', 43, 'RPM_right11', 44, 'RPM_right12Out', 45);

interp_point_1  = u(variable_indices.wing_alpha);
interp_point_2  = u(variable_indices.wing_beta);
interp_point_3  = u(variable_indices.U);
interp_point_4  = u(variable_indices.wing_RPM);
interp_point_5  = u(variable_indices.wing_prop_alpha);
interp_point_6  = u(variable_indices.wing_prop_beta);

end

% y = [U, alpha, beta, p, q, r, wing_alpha, wing_beta, wing_RPM, left_alpha, right_alpha, left_beta, right_beta, wing_prop_alpha, wing_prop_beta, ...
    % tail_alpha, tail_beta, tail_RPM, tailLeft_alpha, tailRight_alpha, tailLeft_beta, tailRight_beta, tail_prop_alpha, ...
    % tail_prop_beta, Q, aileron, elevator, flap, rudder, wing_tilt, tail_tilt, RPM_tailLeft, RPM_tailRight, RPM_leftOut1, RPM_left2, ...
    % RPM_left3, RPM_left4, RPM_left5, RPM_left6In, RPM_right7In, RPM_right8, RPM_right9, RPM_right10, RPM_right11, RPM_right12Out];

== matlab function BechamoNasaOpenModels/Mavrik v1/Mavrik Aero/Cz/CZ_wing_damp_p ==
  data: u input size=[1 45]; interp_point_1 output; interp_point_2 output; interp_point_3 output; interp_point_4 output; interp_point_5 output; interp_point_6 output
function [interp_point_1, interp_point_2, interp_point_3, interp_point_4, interp_point_5, interp_point_6] = fcn(u)

% Find Interpolation Points
variable_indices = struct('U', 1, 'alpha', 2, 'beta', 3, 'p', 4, 'q', 5, 'r', 6, 'wing_alpha', 7, 'wing_beta', 8, 'wing_RPM', 9, 'left_alpha', 10,...
    'right_alpha', 11, 'left_beta', 12, 'right_beta', 13, 'wing_prop_alpha', 14, 'wing_prop_beta', 15, 'tail_alpha', 16, 'tail_beta', 17, 'tail_RPM', 18, 'tailLeft_alpha', 19, 'tailRight_alpha', 20,...
    'tailLeft_beta', 21, 'tailRight_beta', 22, 'tail_prop_alpha', 23, 'tail_prop_beta', 24, 'Q', 25, 'aileron', 26, 'elevator', 27, 'flap', 28, 'rudder', 29, 'wing_tilt', 30,...
    'tail_tilt', 31, 'RPM_tailLeft', 32, 'RPM_tailRight', 33, 'RPM_leftOut1', 34, 'RPM_left2', 35, 'RPM_left3', 36, 'RPM_left4', 37, 'RPM_left5', 38, 'RPM_left6In', 39, 'RPM_right7In', 40,...
    'RPM_right8', 41, 'RPM_right9', 42, 'RPM_right10', 43, 'RPM_right11', 44, 'RPM_right12Out', 45);

interp_point_1  = u(variable_indices.wing_alpha);
interp_point_2  = u(variable_indices.wing_beta);
interp_point_3  = u(variable_indices.U);
interp_point_4  = u(variable_indices.wing_RPM);
interp_point_5  = u(variable_indices.wing_prop_alpha);
interp_point_6  = u(variable_indices.wing_prop_beta);

end

% y = [U, alpha, beta, p, q, r, wing_alpha, wing_beta, wing_RPM, left_alpha, right_alpha, left_beta, right_beta, wing_prop_alpha, wing_prop_beta, ...
    % tail_alpha, tail_beta, tail_RPM, tailLeft_alpha, tailRight_alpha, tailLeft_beta, tailRight_beta, tail_prop_alpha, ...
    % tail_prop_beta, Q, aileron, elevator, flap, rudder, wing_tilt, tail_tilt, RPM_tailLeft, RPM_tailRight, RPM_leftOut1, RPM_left2, ...
    % RPM_left3, RPM_left4, RPM_left5, RPM_left6In, RPM_right7In, RPM_right8, RPM_right9, RPM_right10, RPM_right11, RPM_right12Out];

== matlab function BechamoNasaOpenModels/Mavrik v1/Mavrik Aero/Cz/CZ_wing_damp_q ==
  data: u input size=[1 45]; interp_point_1 output; interp_point_2 output; interp_point_3 output; interp_point_4 output; interp_point_5 output; interp_point_6 output
function [interp_point_1, interp_point_2, interp_point_3, interp_point_4, interp_point_5, interp_point_6] = fcn(u)

% Find Interpolation Points
variable_indices = struct('U', 1, 'alpha', 2, 'beta', 3, 'p', 4, 'q', 5, 'r', 6, 'wing_alpha', 7, 'wing_beta', 8, 'wing_RPM', 9, 'left_alpha', 10,...
    'right_alpha', 11, 'left_beta', 12, 'right_beta', 13, 'wing_prop_alpha', 14, 'wing_prop_beta', 15, 'tail_alpha', 16, 'tail_beta', 17, 'tail_RPM', 18, 'tailLeft_alpha', 19, 'tailRight_alpha', 20,...
    'tailLeft_beta', 21, 'tailRight_beta', 22, 'tail_prop_alpha', 23, 'tail_prop_beta', 24, 'Q', 25, 'aileron', 26, 'elevator', 27, 'flap', 28, 'rudder', 29, 'wing_tilt', 30,...
    'tail_tilt', 31, 'RPM_tailLeft', 32, 'RPM_tailRight', 33, 'RPM_leftOut1', 34, 'RPM_left2', 35, 'RPM_left3', 36, 'RPM_left4', 37, 'RPM_left5', 38, 'RPM_left6In', 39, 'RPM_right7In', 40,...
    'RPM_right8', 41, 'RPM_right9', 42, 'RPM_right10', 43, 'RPM_right11', 44, 'RPM_right12Out', 45);

interp_point_1  = u(variable_indices.wing_alpha);
interp_point_2  = u(variable_indices.wing_beta);
interp_point_3  = u(variable_indices.U);
interp_point_4  = u(variable_indices.wing_RPM);
interp_point_5  = u(variable_indices.wing_prop_alpha);
interp_point_6  = u(variable_indices.wing_prop_beta);

end

% y = [U, alpha, beta, p, q, r, wing_alpha, wing_beta, wing_RPM, left_alpha, right_alpha, left_beta, right_beta, wing_prop_alpha, wing_prop_beta, ...
    % tail_alpha, tail_beta, tail_RPM, tailLeft_alpha, tailRight_alpha, tailLeft_beta, tailRight_beta, tail_prop_alpha, ...
    % tail_prop_beta, Q, aileron, elevator, flap, rudder, wing_tilt, tail_tilt, RPM_tailLeft, RPM_tailRight, RPM_leftOut1, RPM_left2, ...
    % RPM_left3, RPM_left4, RPM_left5, RPM_left6In, RPM_right7In, RPM_right8, RPM_right9, RPM_right10, RPM_right11, RPM_right12Out];

== matlab function BechamoNasaOpenModels/Mavrik v1/Mavrik Aero/Cz/CZ_wing_damp_r ==
  data: u input size=[1 45]; interp_point_1 output; interp_point_2 output; interp_point_3 output; interp_point_4 output; interp_point_5 output; interp_point_6 output
function [interp_point_1, interp_point_2, interp_point_3, interp_point_4, interp_point_5, interp_point_6] = fcn(u)

% Find Interpolation Points
variable_indices = struct('U', 1, 'alpha', 2, 'beta', 3, 'p', 4, 'q', 5, 'r', 6, 'wing_alpha', 7, 'wing_beta', 8, 'wing_RPM', 9, 'left_alpha', 10,...
    'right_alpha', 11, 'left_beta', 12, 'right_beta', 13, 'wing_prop_alpha', 14, 'wing_prop_beta', 15, 'tail_alpha', 16, 'tail_beta', 17, 'tail_RPM', 18, 'tailLeft_alpha', 19, 'tailRight_alpha', 20,...
    'tailLeft_beta', 21, 'tailRight_beta', 22, 'tail_prop_alpha', 23, 'tail_prop_beta', 24, 'Q', 25, 'aileron', 26, 'elevator', 27, 'flap', 28, 'rudder', 29, 'wing_tilt', 30,...
    'tail_tilt', 31, 'RPM_tailLeft', 32, 'RPM_tailRight', 33, 'RPM_leftOut1', 34, 'RPM_left2', 35, 'RPM_left3', 36, 'RPM_left4', 37, 'RPM_left5', 38, 'RPM_left6In', 39, 'RPM_right7In', 40,...
    'RPM_right8', 41, 'RPM_right9', 42, 'RPM_right10', 43, 'RPM_right11', 44, 'RPM_right12Out', 45);

interp_point_1  = u(variable_indices.wing_alpha);
interp_point_2  = u(variable_indices.wing_beta);
interp_point_3  = u(variable_indices.U);
interp_point_4  = u(variable_indices.wing_RPM);
interp_point_5  = u(variable_indices.wing_prop_alpha);
interp_point_6  = u(variable_indices.wing_prop_beta);

end

% y = [U, alpha, beta, p, q, r, wing_alpha, wing_beta, wing_RPM, left_alpha, right_alpha, left_beta, right_beta, wing_prop_alpha, wing_prop_beta, ...
    % tail_alpha, tail_beta, tail_RPM, tailLeft_alpha, tailRight_alpha, tailLeft_beta, tailRight_beta, tail_prop_alpha, ...
    % tail_prop_beta, Q, aileron, elevator, flap, rudder, wing_tilt, tail_tilt, RPM_tailLeft, RPM_tailRight, RPM_leftOut1, RPM_left2, ...
    % RPM_left3, RPM_left4, RPM_left5, RPM_left6In, RPM_right7In, RPM_right8, RPM_right9, RPM_right10, RPM_right11, RPM_right12Out];

== matlab function BechamoNasaOpenModels/Mavrik v1/Mavrik Aero/L/Cl_aileron_wing ==
  data: u input size=[1 45]; interp_point_1 output; interp_point_2 output; interp_point_3 output; interp_point_4 output; interp_point_5 output; interp_point_6 output; interp_point_7 output
function [interp_point_1, interp_point_2, interp_point_3, interp_point_4, interp_point_5, interp_point_6, interp_point_7] = fcn(u)

% Find Interpolation Points
variable_indices = struct('U', 1, 'alpha', 2, 'beta', 3, 'p', 4, 'q', 5, 'r', 6, 'wing_alpha', 7, 'wing_beta', 8, 'wing_RPM', 9, 'left_alpha', 10,...
    'right_alpha', 11, 'left_beta', 12, 'right_beta', 13, 'wing_prop_alpha', 14, 'wing_prop_beta', 15, 'tail_alpha', 16, 'tail_beta', 17, 'tail_RPM', 18, 'tailLeft_alpha', 19, 'tailRight_alpha', 20,...
    'tailLeft_beta', 21, 'tailRight_beta', 22, 'tail_prop_alpha', 23, 'tail_prop_beta', 24, 'Q', 25, 'aileron', 26, 'elevator', 27, 'flap', 28, 'rudder', 29, 'wing_tilt', 30,...
    'tail_tilt', 31, 'RPM_tailLeft', 32, 'RPM_tailRight', 33, 'RPM_leftOut1', 34, 'RPM_left2', 35, 'RPM_left3', 36, 'RPM_left4', 37, 'RPM_left5', 38, 'RPM_left6In', 39, 'RPM_right7In', 40,...
    'RPM_right8', 41, 'RPM_right9', 42, 'RPM_right10', 43, 'RPM_right11', 44, 'RPM_right12Out', 45);

interp_point_1  = u(variable_indices.wing_alpha);
interp_point_2  = u(variable_indices.wing_beta);
interp_point_3  = u(variable_indices.U);
interp_point_4  = u(variable_indices.wing_RPM);
interp_point_5  = u(variable_indices.wing_prop_alpha);
interp_point_6  = u(variable_indices.wing_prop_beta);
interp_point_7  = u(variable_indices.aileron);

end

% y = [U, alpha, beta, p, q, r, wing_alpha, wing_beta, wing_RPM, left_alpha, right_alpha, left_beta, right_beta, wing_prop_alpha, wing_prop_beta, ...
    % tail_alpha, tail_beta, tail_RPM, tailLeft_alpha, tailRight_alpha, tailLeft_beta, tailRight_beta, tail_prop_alpha, ...
    % tail_prop_beta, Q, aileron, elevator, flap, rudder, wing_tilt, tail_tilt, RPM_tailLeft, RPM_tailRight, RPM_leftOut1, RPM_left2, ...
    % RPM_left3, RPM_left4, RPM_left5, RPM_left6In, RPM_right7In, RPM_right8, RPM_right9, RPM_right10, RPM_right11, RPM_right12Out];
